simulink model "PMSM_PR"  (R2023b)
settings: Solver=ode23tb  StartTime=0.0  StopTime=0.4  FixedStep=Ts  RelTol=1e-4  EnableMultiTasking=on
InitFcn:
  | Ts = 1e-6;
  | 
  | Ld=5.25e-3;
  | Lq=12e-3;
undefined symbols (not defined in the file or in its folder): DiscIntNeverNeededParam
libraries: spsDCVoltageSourceLib x1, spsUniversalBridgeLib x1, spsPermanentMagnetSynchronousMachineLib x1, simulink x1, spspowerguiLib x1
settings Model: Creator=Administrator  LastModifiedBy=Guoguo
settings SolverCC: AlgebraicLoopSolver=TrustRegion
settings DataIOCC: LimitDataPoints=on  SaveFormat=Array  SignalLoggingSaveFormat=ModelDataLogs  ReturnWorkspaceOutputs=off
settings OptimizationCC: ExpressionDepthLimit=2147483647  InitFltsAndDblsToZero=on  LifeSpan=inf
settings DebuggingCC: SaveWithParameterizedLinksMsg=none  UnderspecifiedInitializationDetection=Classic  MergeDetectMultiDrivingBlocksExec=none  SolverPrmCheckMsg=warning  FcnCallInpInsideContextMsg=warning  UnconnectedInputMsg=warning  UnconnectedOutputMsg=warning  UnconnectedLineMsg=warning  StateNameClashWarn=warning  SFUnexpectedBacktrackingDiag=warning  SFNoUnconditionalDefaultTransitionDiag=warning  SFExecutionAtInitializationDiag=none  ArithmeticOperatorsInVariantConditions=warning
settings HardwareCC: ProdBitPerPointer=32  ProdBitPerSizeT=32  ProdBitPerPtrDiffT=32  ProdLargestAtomicFloat=None  ProdIntDivRoundTo=Undefined  ProdEndianess=Unspecified  ProdWordSize=32  ProdHWDeviceType=32-bit Generic
settings ModelReferenceCC: EnableRefExpFcnMdlSchedulingChecks=on  PropagateSignalLabelsOutOfModel=off
settings SFSimCC: SimUseLocalCustomCode=off  CustomCodeUndefinedFunction=UseInterfaceOnly
settings RTWCC: RTWUseLocalCustomCode=off
settings CodeAppCC: StateflowObjectComments=on
settings GRTTargetCC: TargetFcnLib=ansi_tfl_tmw.mat  TargetLangStandard=C89/C90 (ANSI)  CombineOutputUpdateFcns=off  GRTInterface=on
settings ConfigComp: CovMetricSettings=dw  CovSaveCumulativeToWorkspaceVar=on  CovSaveSingleToWorkspaceVar=on  CovExternalEMLEnable=off  CovSFcnEnable=off
settings SimscapeCC: SimscapeNormalizeSystem=off

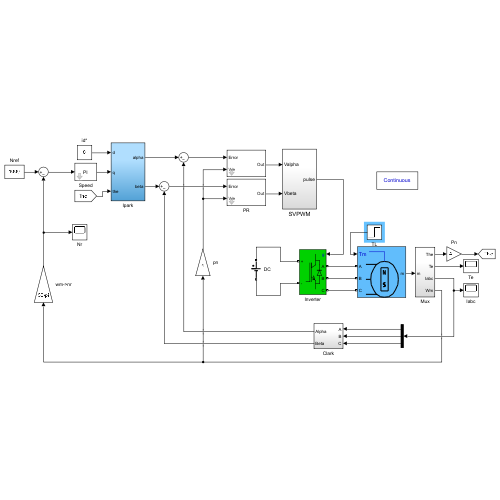
[thumbnail: Simulink's stored preview of the top-level diagram]
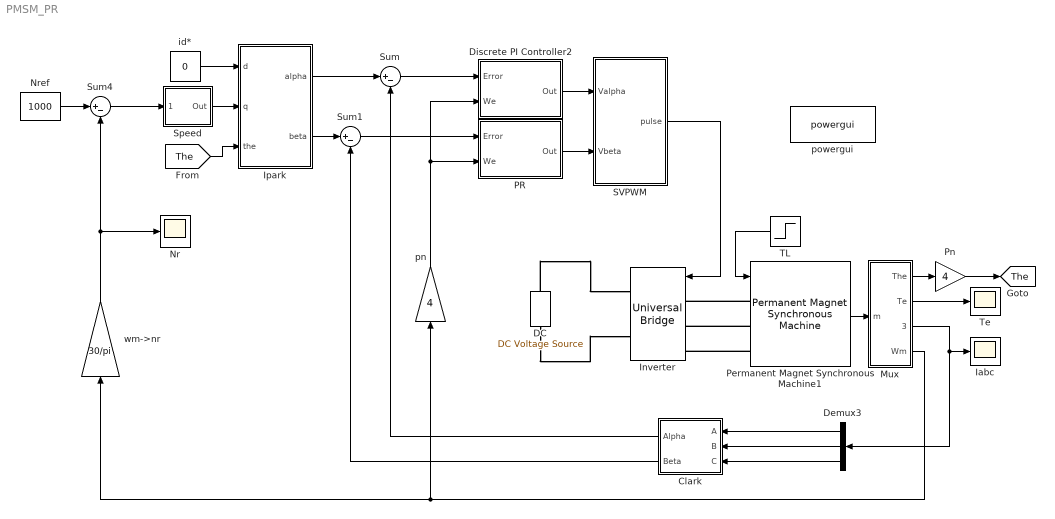
== system PMSM_PR ==
  Clark : Subsystem
  "DC " : spsDCVoltageSourceLib/DC Voltage Source  Amplitude=311  Measurements=None
  Demux3 : Demux  Outputs=3
  Discrete PI Controller2 : Subsystem  AncestorBlock=|  DialogController=POWERSYS.PowerSysDialog  mask(Discrete PI Controller){Kp=100, wc=200, ki=1000, Par_Limits=[300/sqrt(3) -300/sqrt(3)], Init=0, Ts=Ts}
      | powerlib_extras/Discrete 
      | Control Blocks/Discrete
      | PI Controller
      mask prompts: Kp "Proportional gain (Kp):"; wc "Cut-off frequency(wc)"; ki "PR integral gain (ki)"; Par_Limits "Output limits: [ Upper   Lower ]"; Init "Output initial value:"; Ts "Sample time:"
      mask help: This block implements a discrete PI controller.
      mask init:
      | UpperLimit=Par_Limits(1);
      | LowerLimit=Par_Limits(2);
      | power_initmask();
      mask Help: This block is part of a subset of blocks in the Extras library that does not have documentation associated with it, other than the block mask description.
  Iabc : Scope
  Inverter : spsUniversalBridgeLib/Universal Bridge  Arms=3  SnubberResistance=1e5  SnubberCapacitance=inf  Device=IGBT / Diodes  Ron=1e-3  Lon=0  ForwardVoltages="[  0  0  ]"  ForwardVoltage=0  GTOparameters=[ 10e-6 , 20e-6 ]  IGBTparameters=[ 1e-6 , 2e-6 ]  Measurements=None  Measurements_2=None  converterType=Rectifier
  Ipark : Subsystem
  Mux : Subsystem
  Nr : Scope
  Nref : Constant  Value=1000
  PR : Subsystem  AncestorBlock=|  DialogController=POWERSYS.PowerSysDialog  mask(Discrete PI Controller){Kp=100, wc=200, ki=1000, Par_Limits=[300/sqrt(3) -300/sqrt(3)], Init=0, Ts=Ts}
      | powerlib_extras/Discrete 
      | Control Blocks/Discrete
      | PI Controller
      mask prompts: Kp "Proportional gain (Kp):"; wc "Cut-off frequency(wc)"; ki "PR integral gain (ki)"; Par_Limits "Output limits: [ Upper   Lower ]"; Init "Output initial value:"; Ts "Sample time:"
      mask help: This block implements a discrete PI controller.
      mask init:
      | UpperLimit=Par_Limits(1);
      | LowerLimit=Par_Limits(2);
      | power_initmask();
      mask Help: This block is part of a subset of blocks in the Extras library that does not have documentation associated with it, other than the block mask description.
  Permanent Magnet Synchronous Machine1 : spsPermanentMagnetSynchronousMachineLib/Permanent Magnet Synchronous Machine  NbPhases=3  FluxDistribution=Sinusoidal  RotorType=Salient-pole  MechanicalLoad=Torque Tm  PresetModel=No  ShowDetailedParameters=on  MeasurementBus=off  Resistance=0.958  Inductance=8.5e-3  dqInductances=[5.25e-3,12e-3]  La=0.000835  MachineConstant=Flux linkage established by magnets (V.s)  Flux=0.1827  VoltageCst=132.5525  TorqueCst=1.0962  Flat=120  Mechanical=[0.003 0.008 4]  PolePairs=3  InitialConditions=[0,0, 0,0]  InitialConditions5ph=[0 0 0 0 0 0]  RefAngle=Aligned with phase A axis (original Park)  IterativeDiscreteModel=Trapezoidal non iterative  TsBlock=-1  TsPowergui=0
  Pn : Gain  Gain=4
  SVPWM : Subsystem
  Speed : Subsystem  AncestorBlock=|  DialogController=POWERSYS.PowerSysDialog  mask(Discrete PI Controller){Kpw=0.08, Kiw=4, Ba=0, Par_Limits=[20 -20], Init=0, Ts=Ts}
      | powerlib_extras/Discrete 
      | Control Blocks/Discrete
      | PI Controller
      mask prompts: Kpw "Proportional gain (Kp):"; Kiw "Integral gain (Ki):"; Ba "feedback gain (Ba)"; Par_Limits "Output limits: [ Upper   Lower ]"; Init "Output initial value:"; Ts "Sample time:"
      mask help: This block implements a discrete PI controller.
      mask init:
      | UpperLimit=Par_Limits(1);
      | LowerLimit=Par_Limits(2);
      | power_initmask();
      mask Help: This block is part of a subset of blocks in the Extras library that does not have documentation associated with it, other than the block mask description.
      mask Display: disp('PI');
  Sum : Sum  Inputs=|+-
  Sum1 : Sum  Inputs=|+-
  Sum4 : Sum  Inputs=|+-
  TL : Step  Time=0.2  After=10  SampleTime=0
  Te : Scope
  id* : Constant  Value=0
  pn : Gain  Gain=4
  powergui : spspowerguiLib/powergui  SimulationMode=Continuous  SampleTime=Ts  frequency=60  Iterations=50  frequencyindice=0  Pbase=100e6  ErrMax=1e-4  UnitsV=kV  UnitsW=MW  buscounter=0  FunctionMessages=off  echomessages=off  EnableUseOfTLC=off  CurrentSourceSwitches=on  DisableSnubberDevices=off  DisableRonSwitches=off  DisableVfSwitches=off  DisplayEquations=off  AutomaticDiscreteSolvers=off  SolverType=Tustin/Backward Euler (TBE)  Interpol=off  ExternalGateDelay=off  methode=off  Ts=0  x0status=blocks  SPID=off  SwTol=0  HookPort=off  NonlinearTolerance=1e-4  nMaxIteration=100  ContinueOnMaxIteration=off  RestoreLinks=warning  ResistiveCurrentMeasurement=off  Frange=[0:2:500]  Ylog=off  Xlog=on  ShowGrid=off  save=off  variable=ZData  structure=0  ZoomFFT=off  StartTime=0.0  cycles=1  DisplayStyle=1  fundamental=60  FreqAxis=off  MaxFrequency=1000  frequencyindicesteady=1  RmsSteady=1  display=off
  wm->nr : Gain  Gain=30/pi
  tag scope: The=global
  wires:
  SVPWM/1(pulse) -> Inverter/1
  Permanent Magnet Synchronous Machine1/1 -> Mux/1(m)
  Mux/1(The) -> Pn/1
  Mux/3(Iabc) -> Demux3/1, Iabc/1
  Mux/2(Te) -> Te/1
  Demux3/1 -> Clark/1(A)
  Demux3/2 -> Clark/2(B)
  Demux3/3 -> Clark/3(C)
  TL/1 -> Permanent Magnet Synchronous Machine1/1
  Sum1/1 -> PR/1(Error)
  Sum/1 -> Discrete PI Controller2/1(Error)
  Sum4/1 -> Speed/1(Error)
  Ipark/1(alpha) -> Sum/1
  id*/1 -> Ipark/1(d)
  Speed/1(Out) -> Ipark/2(q)
  Ipark/2(beta) -> Sum1/1
  Mux/4(Wm) -> pn/1, wm->nr/1
  Nref/1 -> Sum4/1
  wm->nr/1 -> Sum4/2, Nr/1
  PR/1(Out) -> SVPWM/2(Vbeta)
  Discrete PI Controller2/1(Out) -> SVPWM/1(Valpha)
  Clark/1(Alpha) -> Sum/2
  Clark/2(Beta) -> Sum1/2
  pn/1 -> Discrete PI Controller2/2(We), PR/2(We)
  Pn/1 -> [The]
  [The] -> Ipark/3(the)
  connections:
  "DC "/RConn1 -- Inverter/RConn1
  "DC "/LConn1 -- Inverter/RConn2
  Permanent Magnet Synchronous Machine1/LConn1 -- Inverter/LConn1
  Permanent Magnet Synchronous Machine1/LConn2 -- Inverter/LConn2
  Permanent Magnet Synchronous Machine1/LConn3 -- Inverter/LConn3

== system PMSM_PR/Clark ==
  A : Inport
  B : Inport  Port=2
  C : Inport  Port=3
  Mux : Mux  Inputs=3
  alpha : Fcn  Expr=(u(1)-0.5*(u(2)+u(3)))*2/3
  beta : Fcn  Expr=sqrt(3)/2*(u(2)-u(3))*2/3
  Alpha : Outport
  Beta : Outport  Port=2
  wires:
  alpha/1 -> Alpha/1
  B/1 -> Mux/2
  C/1 -> Mux/3
  A/1 -> Mux/1
  Mux/1 -> beta/1, alpha/1
  beta/1 -> Beta/1

== system PMSM_PR/Discrete PI Controller2 ==
  note: Discrete PID Controller
  note: Pierre Giroux, Gilbert Sybille
      | Power System Simulation Laboratory
      | IREQ, Hydro-Quebc
  Error : Inport  SampleTime=Ts
  We : Inport  Port=2  SampleTime=Ts
  Kp4 : Gain  Gain=Kp  SaturateOnIntegerOverflow=on  SampleTime=Ts  OutDataTypeStr=Inherit: Same as input  ParamDataTypeStr=Inherit: Same as input
  R : Subsystem
  Sum6 : Sum  InputSameDT=on  SaturateOnIntegerOverflow=on  SampleTime=Ts  OutDataTypeStr=Inherit: Same as first input
  Zero-Order Hold : ZeroOrderHold  SampleTime=Ts
  Out : Outport  SampleTime=Ts  InitialOutput=0
  wires:
  Zero-Order Hold/1 -> Sum6/1
  We/1 -> R/2(we)
  Sum6/1 -> Out/1
  Kp4/1 -> Zero-Order Hold/1
  Error/1 -> Kp4/1, R/1(error)
  R/1(Out) -> Sum6/2

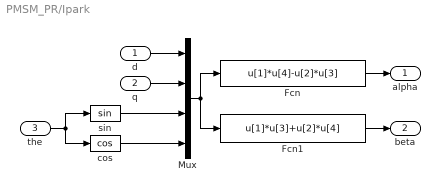
== system PMSM_PR/Ipark ==
  d : Inport
  q : Inport  Port=2
  the : Inport  Port=3
  Fcn : Fcn  Expr=u[1]*u[4]-u[2]*u[3]
  Fcn1 : Fcn  Expr=u[1]*u[3]+u[2]*u[4]
  Mux : Mux
  cos : Trigonometry  Operator=cos
  sin : Trigonometry
  alpha : Outport
  beta : Outport  Port=2
  wires:
  d/1 -> Mux/1
  q/1 -> Mux/2
  Mux/1 -> Fcn1/1, Fcn/1
  sin/1 -> Mux/3
  cos/1 -> Mux/4
  the/1 -> sin/1, cos/1
  Fcn/1 -> alpha/1
  Fcn1/1 -> beta/1

== system PMSM_PR/Mux ==
  m : Inport
  Bus Selector : BusSelector  OutputSignals=Stator current is_a (A),Stator current is_b (A),Stator current is_c (A)
  Bus Selector1 : BusSelector  OutputSignals=Rotor speed wm (rad/s),Rotor angle thetam (rad),Electromagnetic torque Te (N*m)
  Mux : Mux  Inputs=3
  The : Outport
  Te : Outport  Port=2
  Iabc : Outport  Port=3
  Wm : Outport  Port=4
  wires:
  Bus Selector1/1 -> Wm/1  "<Rotor speed wm (rad/s)>"
  Bus Selector1/2 -> The/1  "<Rotor angle thetam (rad)>"
  Bus Selector1/3 -> Te/1  "<Electromagnetic torque Te (N*m)>"
  m/1 -> Bus Selector/1, Bus Selector1/1
  Bus Selector/2 -> Mux/2  "<Stator current is_b (A)>"
  Bus Selector/3 -> Mux/3  "<Stator current is_c (A)>"
  Bus Selector/1 -> Mux/1  "<Stator current is_a (A)>"
  Mux/1 -> Iabc/1

== system PMSM_PR/PR ==
  note: Pierre Giroux, Gilbert Sybille
      | Power System Simulation Laboratory
      | IREQ, Hydro-Quebc
  note: Discrete PID Controller
  Error : Inport  SampleTime=Ts
  We : Inport  Port=2  SampleTime=Ts
  Kp4 : Gain  Gain=Kp  SaturateOnIntegerOverflow=on  SampleTime=Ts  OutDataTypeStr=Inherit: Same as input  ParamDataTypeStr=Inherit: Same as input
  R : Subsystem
  Sum6 : Sum  InputSameDT=on  SaturateOnIntegerOverflow=on  SampleTime=Ts  OutDataTypeStr=Inherit: Same as first input
  Zero-Order Hold : ZeroOrderHold  SampleTime=Ts
  Out : Outport  SampleTime=Ts  InitialOutput=0
  wires:
  R/1(Out) -> Sum6/2
  Error/1 -> R/1(error), Kp4/1
  Kp4/1 -> Zero-Order Hold/1
  Sum6/1 -> Out/1
  We/1 -> R/2(we)
  Zero-Order Hold/1 -> Sum6/1

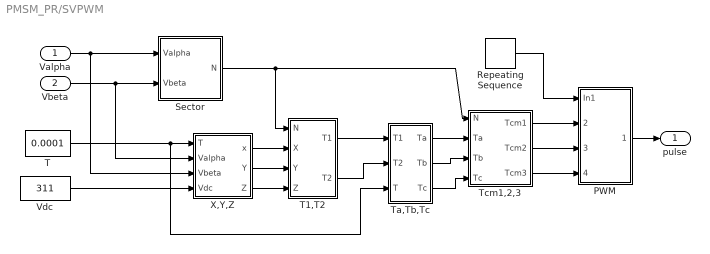
== system PMSM_PR/SVPWM ==
  Valpha : Inport
  Vbeta : Inport  Port=2
  PWM : Subsystem
  Repeating Sequence : simulink/Sources/Repeating Sequence  rep_seq_t=[0 0.00005 0.0001]  rep_seq_y=[0 0.00005 0]
  Sector : Subsystem
  T : Constant  Value=0.0001
  T1,T2 : Subsystem
  Ta,Tb,Tc : Subsystem
  Tcm1,2,3 : Subsystem
  Vdc : Constant  Value=311
  X,Y,Z : Subsystem
  pulse : Outport
  wires:
  PWM/1(PWM) -> pulse/1
  Repeating Sequence/1 -> PWM/1(In1)
  Tcm1,2,3/3(Tcm3) -> PWM/4(Tcm3)
  Tcm1,2,3/2(Tcm2) -> PWM/3(Tcm2)
  Tcm1,2,3/1(Tcm1) -> PWM/2(Tcm1)
  Ta,Tb,Tc/3(Tc) -> Tcm1,2,3/4(Tc)
  Ta,Tb,Tc/2(Tb) -> Tcm1,2,3/3(Tb)
  Ta,Tb,Tc/1(Ta) -> Tcm1,2,3/2(Ta)
  T1,T2/2(T2) -> Ta,Tb,Tc/2(T2)
  T1,T2/1(T1) -> Ta,Tb,Tc/1(T1)
  X,Y,Z/3(Z) -> T1,T2/4(Z)
  X,Y,Z/2(Y) -> T1,T2/3(Y)
  X,Y,Z/1(x) -> T1,T2/2(X)
  Sector/1(N) -> T1,T2/1(N), Tcm1,2,3/1(N)
  Vdc/1 -> X,Y,Z/4(Vdc)
  T/1 -> Ta,Tb,Tc/3(T), X,Y,Z/1(T)
  Vbeta/1 -> X,Y,Z/2(Valpha), Sector/2(Vbeta)
  Valpha/1 -> X,Y,Z/3(Vbeta), Sector/1(Valpha)

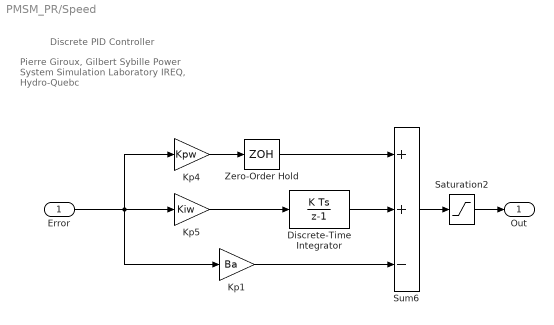
== system PMSM_PR/Speed ==
  note: Discrete PID Controller
  note: Pierre Giroux, Gilbert Sybille
      | Power System Simulation Laboratory
      | IREQ, Hydro-Quebc
  Error : Inport  SampleTime=Ts
  Discrete-Time Integrator : DiscreteIntegrator  InitialCondition=Init  SampleTime=Ts  LimitOutput=on  UpperSaturationLimit=UpperLimit  LowerSaturationLimit=LowerLimit  ICPrevOutput=DiscIntNeverNeededParam  ICPrevScaledInput=DiscIntNeverNeededParam
  Kp1 : Gain  Gain=Ba  SaturateOnIntegerOverflow=on  SampleTime=Ts  OutDataTypeStr=Inherit: Same as input  ParamDataTypeStr=Inherit: Same as input
  Kp4 : Gain  Gain=Kpw  SaturateOnIntegerOverflow=on  SampleTime=Ts  OutDataTypeStr=Inherit: Same as input  ParamDataTypeStr=Inherit: Same as input
  Kp5 : Gain  Gain=Kiw  SaturateOnIntegerOverflow=on  SampleTime=Ts  OutDataTypeStr=Inherit: Same as input  ParamDataTypeStr=Inherit: Same as input
  Saturation2 : Saturate  UpperLimit=UpperLimit  LowerLimit=LowerLimit  SampleTime=Ts
  Sum6 : Sum  Inputs=++-  InputSameDT=on  SaturateOnIntegerOverflow=on  SampleTime=Ts  OutDataTypeStr=Inherit: Same as first input
  Zero-Order Hold : ZeroOrderHold  SampleTime=Ts
  Out : Outport  SampleTime=Ts  InitialOutput=0
  wires:
  Error/1 -> Kp1/1, Kp5/1, Kp4/1
  Zero-Order Hold/1 -> Sum6/1
  Saturation2/1 -> Out/1
  Discrete-Time Integrator/1 -> Sum6/2
  Kp4/1 -> Zero-Order Hold/1
  Kp5/1 -> Discrete-Time Integrator/1
  Sum6/1 -> Saturation2/1
  Kp1/1 -> Sum6/3

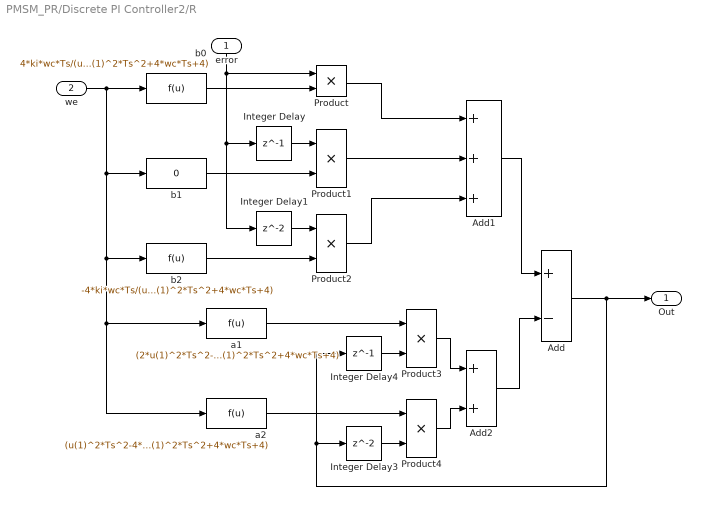
== system PMSM_PR/Discrete PI Controller2/R ==
  error : Inport
  we : Inport  Port=2
  Add : Sum  Inputs=+-
  Add1 : Sum  Inputs=+++
  Add2 : Sum
  Integer Delay : Delay  DelayLength=1  SampleTime=Ts
  Integer Delay1 : Delay  SampleTime=Ts
  Integer Delay3 : Delay
  Integer Delay4 : Delay  DelayLength=1  SampleTime=Ts
  Product{,1..4} (5 alike) : Product  RndMeth=Zero
  a1 : Fcn  Expr=(2*u(1)^2*Ts^2-8)/(u(1)^2*Ts^2+4*wc*Ts+4)  SampleTime=Ts
  a2 : Fcn  Expr=(u(1)^2*Ts^2-4*wc*Ts+4)/(u(1)^2*Ts^2+4*wc*Ts+4)  SampleTime=Ts
  b0 : Fcn  Expr=4*ki*wc*Ts/(u(1)^2*Ts^2+4*wc*Ts+4)
  b1 : Fcn  Expr=0
  b2 : Fcn  Expr=-4*ki*wc*Ts/(u(1)^2*Ts^2+4*wc*Ts+4)
  Out : Outport
  wires:
  we/1 -> b0/1, b1/1, b2/1, a1/1, a2/1
  b0/1 -> Product/2
  b1/1 -> Product1/2
  Integer Delay/1 -> Product1/1
  Integer Delay1/1 -> Product2/1
  b2/1 -> Product2/2
  Product/1 -> Add1/1
  Product1/1 -> Add1/2
  Product2/1 -> Add1/3
  Add/1 -> Out/1, Integer Delay3/1, Integer Delay4/1
  a1/1 -> Product3/1
  a2/1 -> Product4/1
  Integer Delay3/1 -> Product4/2
  Integer Delay4/1 -> Product3/2
  error/1 -> Product/1, Integer Delay/1, Integer Delay1/1
  Product4/1 -> Add2/2
  Product3/1 -> Add2/1
  Add2/1 -> Add/2
  Add1/1 -> Add/1

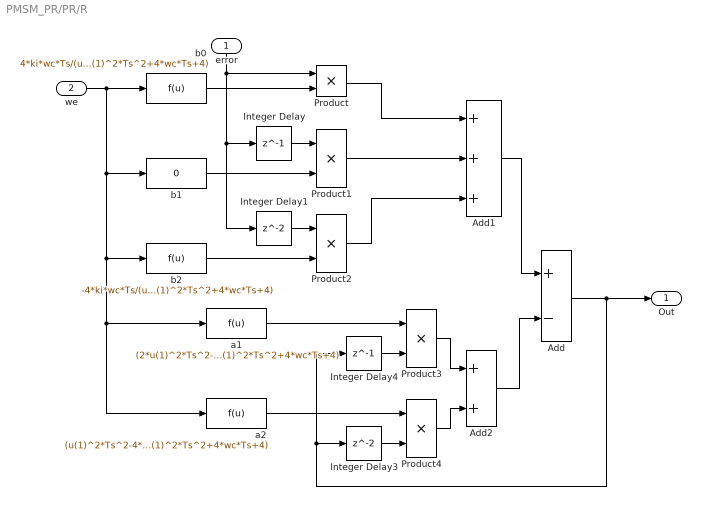
== system PMSM_PR/PR/R ==
  error : Inport
  we : Inport  Port=2
  Add : Sum  Inputs=+-
  Add1 : Sum  Inputs=+++
  Add2 : Sum
  Integer Delay : Delay  DelayLength=1  SampleTime=Ts
  Integer Delay1 : Delay  SampleTime=Ts
  Integer Delay3 : Delay
  Integer Delay4 : Delay  DelayLength=1  SampleTime=Ts
  Product{,1..4} (5 alike) : Product  RndMeth=Zero
  a1 : Fcn  Expr=(2*u(1)^2*Ts^2-8)/(u(1)^2*Ts^2+4*wc*Ts+4)  SampleTime=Ts
  a2 : Fcn  Expr=(u(1)^2*Ts^2-4*wc*Ts+4)/(u(1)^2*Ts^2+4*wc*Ts+4)  SampleTime=Ts
  b0 : Fcn  Expr=4*ki*wc*Ts/(u(1)^2*Ts^2+4*wc*Ts+4)
  b1 : Fcn  Expr=0
  b2 : Fcn  Expr=-4*ki*wc*Ts/(u(1)^2*Ts^2+4*wc*Ts+4)
  Out : Outport
  wires:
  Add1/1 -> Add/1
  Add2/1 -> Add/2
  Product3/1 -> Add2/1
  Product4/1 -> Add2/2
  error/1 -> Integer Delay1/1, Integer Delay/1, Product/1
  Integer Delay4/1 -> Product3/2
  Integer Delay3/1 -> Product4/2
  a2/1 -> Product4/1
  a1/1 -> Product3/1
  Add/1 -> Integer Delay4/1, Integer Delay3/1, Out/1
  Product2/1 -> Add1/3
  Product1/1 -> Add1/2
  Product/1 -> Add1/1
  b2/1 -> Product2/2
  Integer Delay1/1 -> Product2/1
  Integer Delay/1 -> Product1/1
  b1/1 -> Product1/2
  b0/1 -> Product/2
  we/1 -> a2/1, a1/1, b2/1, b1/1, b0/1

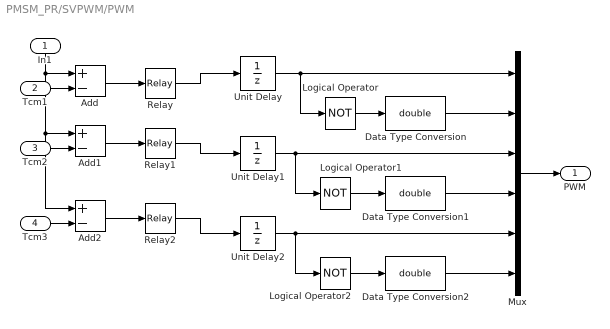
== system PMSM_PR/SVPWM/PWM ==
  In1 : Inport
  Tcm1 : Inport  Port=2
  Tcm2 : Inport  Port=3
  Tcm3 : Inport  Port=4
  Add : Sum  Inputs=+-
  Add1 : Sum  Inputs=+-
  Add2 : Sum  Inputs=+-
  Data Type Conversion : DataTypeConversion  OutDataTypeStr=double  SaturateOnIntegerOverflow=off  RndMeth=Floor
  Data Type Conversion1 : DataTypeConversion  OutDataTypeStr=double  SaturateOnIntegerOverflow=off  RndMeth=Floor
  Data Type Conversion2 : DataTypeConversion  OutDataTypeStr=double  SaturateOnIntegerOverflow=off  RndMeth=Floor
  Logical Operator : Logic  Operator=NOT  AllPortsSameDT=off  OutDataTypeStr=boolean
  Logical Operator1 : Logic  Operator=NOT  AllPortsSameDT=off  OutDataTypeStr=boolean
  Logical Operator2 : Logic  Operator=NOT  AllPortsSameDT=off  OutDataTypeStr=boolean
  Mux : Mux  Inputs=6
  Relay : Relay  OffSwitchValue=-eps
  Relay1 : Relay  OffSwitchValue=-eps
  Relay2 : Relay  OffSwitchValue=-eps
  Unit Delay : UnitDelay  SampleTime=-1  HasFrameUpgradeWarning=on
  Unit Delay1 : UnitDelay  SampleTime=-1  HasFrameUpgradeWarning=on
  Unit Delay2 : UnitDelay  SampleTime=-1  HasFrameUpgradeWarning=on
  PWM : Outport
  wires:
  Tcm3/1 -> Add2/2
  Tcm2/1 -> Add1/2
  Tcm1/1 -> Add/2
  Relay2/1 -> Unit Delay2/1
  Relay1/1 -> Unit Delay1/1
  Relay/1 -> Unit Delay/1
  Unit Delay2/1 -> Mux/5, Logical Operator2/1
  Unit Delay1/1 -> Mux/3, Logical Operator1/1
  Unit Delay/1 -> Logical Operator/1, Mux/1
  Mux/1 -> PWM/1
  Data Type Conversion/1 -> Mux/2
  Data Type Conversion1/1 -> Mux/4
  Data Type Conversion2/1 -> Mux/6
  Logical Operator2/1 -> Data Type Conversion2/1
  Logical Operator1/1 -> Data Type Conversion1/1
  Logical Operator/1 -> Data Type Conversion/1
  Add1/1 -> Relay1/1
  Add2/1 -> Relay2/1
  Add/1 -> Relay/1
  In1/1 -> Add/1, Add2/1, Add1/1

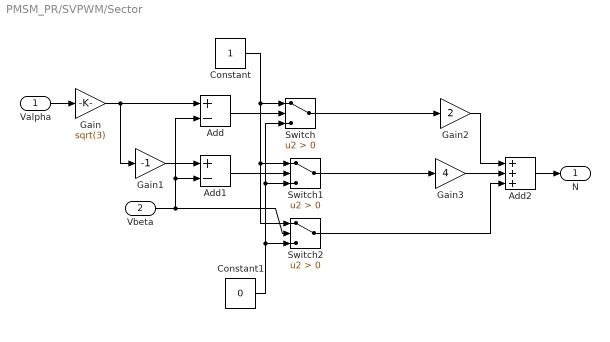
== system PMSM_PR/SVPWM/Sector ==
  Valpha : Inport
  Vbeta : Inport  Port=2
  Add : Sum  Inputs=+-
  Add1 : Sum  Inputs=+-
  Add2 : Sum  Inputs=+++
  Constant : Constant
  Constant1 : Constant  Value=0
  Gain : Gain  Gain=sqrt(3)
  Gain1 : Gain  Gain=-1
  Gain2 : Gain  Gain=2
  Gain3 : Gain  Gain=4
  Switch : Switch  Criteria=u2 > Threshold  SaturateOnIntegerOverflow=off  InputSameDT=off
  Switch1 : Switch  Criteria=u2 > Threshold  SaturateOnIntegerOverflow=off  InputSameDT=off
  Switch2 : Switch  Criteria=u2 > Threshold  SaturateOnIntegerOverflow=off  InputSameDT=off
  N : Outport
  wires:
  Add2/1 -> N/1
  Valpha/1 -> Gain/1
  Gain3/1 -> Add2/2
  Gain2/1 -> Add2/1
  Add1/1 -> Switch1/2
  Gain1/1 -> Add1/1
  Switch1/1 -> Gain3/1
  Switch2/1 -> Add2/3
  Switch/1 -> Gain2/1
  Add/1 -> Switch/2
  Gain/1 -> Gain1/1, Add/1
  Constant1/1 -> Switch/3, Switch1/3, Switch2/3
  Constant/1 -> Switch1/1, Switch2/1, Switch/1
  Vbeta/1 -> Add1/2, Add/2, Switch2/2

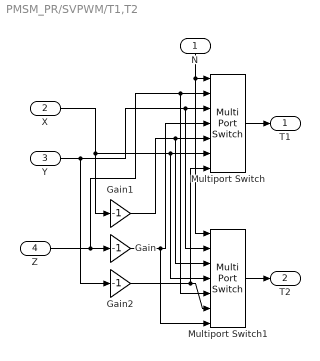
== system PMSM_PR/SVPWM/T1,T2 ==
  N : Inport
  X : Inport  Port=2
  Y : Inport  Port=3
  Z : Inport  Port=4
  Gain : Gain  Gain=-1
  Gain1 : Gain  Gain=-1
  Gain2 : Gain  Gain=-1
  Multiport Switch : MultiPortSwitch  Inputs=6  SaturateOnIntegerOverflow=off  InputSameDT=off
  Multiport Switch1 : MultiPortSwitch  Inputs=6  SaturateOnIntegerOverflow=off  InputSameDT=off
  T1 : Outport
  T2 : Outport  Port=2
  wires:
  Multiport Switch1/1 -> T2/1
  Multiport Switch/1 -> T1/1
  Gain2/1 -> Multiport Switch/7, Multiport Switch1/6
  Gain1/1 -> Multiport Switch1/3, Multiport Switch/5
  X/1 -> Gain1/1, Multiport Switch/6, Multiport Switch1/4
  Gain/1 -> Multiport Switch1/7, Multiport Switch/4
  Y/1 -> Gain2/1, Multiport Switch1/2, Multiport Switch/3
  Z/1 -> Multiport Switch/2, Multiport Switch1/5, Gain/1
  N/1 -> Multiport Switch/1, Multiport Switch1/1

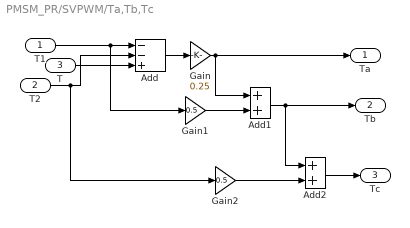
== system PMSM_PR/SVPWM/Ta,Tb,Tc ==
  T1 : Inport
  T2 : Inport  Port=2
  T : Inport  Port=3
  Add : Sum  Inputs=--+
  Add1 : Sum
  Add2 : Sum
  Gain : Gain  Gain=0.25
  Gain1 : Gain  Gain=0.5
  Gain2 : Gain  Gain=0.5
  Ta : Outport
  Tb : Outport  Port=2
  Tc : Outport  Port=3
  wires:
  T/1 -> Add/3
  Add2/1 -> Tc/1
  Gain2/1 -> Add2/2
  Add1/1 -> Add2/1, Tb/1
  Gain1/1 -> Add1/2
  Gain/1 -> Add1/1, Ta/1
  Add/1 -> Gain/1
  T2/1 -> Add/2, Gain2/1
  T1/1 -> Add/1, Gain1/1

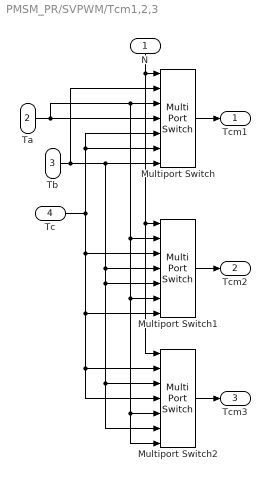
== system PMSM_PR/SVPWM/Tcm1,2,3 ==
  N : Inport
  Ta : Inport  Port=2
  Tb : Inport  Port=3
  Tc : Inport  Port=4
  Multiport Switch : MultiPortSwitch  Inputs=6  SaturateOnIntegerOverflow=off  InputSameDT=off
  Multiport Switch1 : MultiPortSwitch  Inputs=6  SaturateOnIntegerOverflow=off  InputSameDT=off
  Multiport Switch2 : MultiPortSwitch  Inputs=6  SaturateOnIntegerOverflow=off  InputSameDT=off
  Tcm1 : Outport
  Tcm2 : Outport  Port=2
  Tcm3 : Outport  Port=3
  wires:
  Multiport Switch2/1 -> Tcm3/1
  Multiport Switch1/1 -> Tcm2/1
  Multiport Switch/1 -> Tcm1/1
  N/1 -> Multiport Switch2/1, Multiport Switch1/1, Multiport Switch/1
  Tc/1 -> Multiport Switch1/3, Multiport Switch1/7, Multiport Switch2/2, Multiport Switch2/4, Multiport Switch/5, Multiport Switch/6
  Ta/1 -> Multiport Switch/4, Multiport Switch/3, Multiport Switch1/2, Multiport Switch1/6, Multiport Switch2/5, Multiport Switch2/7
  Tb/1 -> Multiport Switch/2, Multiport Switch/7, Multiport Switch1/4, Multiport Switch1/5, Multiport Switch2/3, Multiport Switch2/6

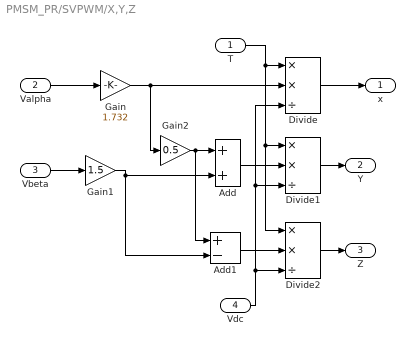
== system PMSM_PR/SVPWM/X,Y,Z ==
  T : Inport
  Valpha : Inport  Port=2
  Vbeta : Inport  Port=3
  Vdc : Inport  Port=4
  Add : Sum
  Add1 : Sum  Inputs=+-
  Divide : Product  Inputs=**/
  Divide1 : Product  Inputs=**/
  Divide2 : Product  Inputs=**/
  Gain : Gain  Gain=1.732
  Gain1 : Gain  Gain=1.5
  Gain2 : Gain  Gain=0.5
  x : Outport
  Y : Outport  Port=2
  Z : Outport  Port=3
  wires:
  Divide2/1 -> Z/1
  Divide1/1 -> Y/1
  Divide/1 -> x/1
  Vbeta/1 -> Gain1/1
  Valpha/1 -> Gain/1
  Add1/1 -> Divide2/2
  Add/1 -> Divide1/2
  Gain1/1 -> Add1/2, Add/2
  Gain2/1 -> Add1/1, Add/1
  Gain/1 -> Gain2/1, Divide/2
  Vdc/1 -> Divide/3, Divide1/3, Divide2/3
  T/1 -> Divide2/1, Divide1/1, Divide/1
